simulink model "Medium_Self_Balance_Vehicle"  (R2021b)
settings: Solver=FixedStepDiscrete  StartTime=0.0  StopTime=10.0  FixedStep=0.005  RelTol=1e-3
libraries: TIMERS_Lib x9, GPIO_Lib x8, REG_Lib x4, ADC_Lib x1, STM32_Config_Lib x1, USART_Lib x1
(part 2 of 2)

== system Medium_Self_Balance_Vehicle/Function-Call Subsystem/Subsystem9/If Action Subsystem5 ==
  Action Port : ActionPort  ActionPortLabel=else { }
  Constant1 : Constant  Value=-1  OutDataTypeStr=int16
  Constant3 : Constant
  Constant4 : Constant  Value=0
  Data Store Read1 : DataStoreRead  DataStoreName=motob  IndexOptions=Index vector (dialog)  Indices=1  OutputSizes=1
  Divide : Product  Inputs=**
  GPIO_Write3 : GPIO_Lib/GPIO_Write  Port_name=GPIOB  Pin0=off  Toggle_Pin0=off  Pin1=off  Toggle_Pin1=off  Pin2=off  Toggle_Pin2=off  Pin3=off  Toggle_Pin3=off  Pin4=off  Toggle_Pin4=off  Pin5=off  Toggle_Pin5=off  Pin6=off  Toggle_Pin6=off  Pin7=off  Toggle_Pin7=off  Pin8=off  Toggle_Pin8=off  Pin9=off  Toggle_Pin9=off  Pin10=off  Toggle_Pin10=off  Pin11=off  Toggle_Pin11=off  Pin12=on  Toggle_Pin12=off  Pin13=on  Toggle_Pin13=off  Pin14=off  Toggle_Pin14=off  Pin15=off  Toggle_Pin15=off  PinList="GPIOA4  15GPIOB3   4   5   8   9  12  13  14  15"
      settings: SourceProductName=Target Support Package - STM32 Adapter
  Timers : TIMERS_Lib/Timers  currentTIM=TIM1  TIM_Name=TIM1  sysUsingTimer=off  TIM_APBClock=72000000  TIM_Set_Clk=off  TIM_Prescaler=0  TIM_Clock=72000000.00  Variable_frequency=off  TIM_Set_OutFreq=off  TIM_ARR=7199  Output_frequency=10001.39  Repetition_counter=0  TIM_Mode=Up  TIM_DMA=none  TIM_IRQ=off  TIM_IRQ_ONLY=off  TIM_UP=off  TIM_TRG=off  TIM_COM=off  TIM_BRK=off  NbTIM=4  CH1_enable=on  CH1N_enable=off  CH1_type=Output_PWM  CH1_DMA=off  CH1_int=off  CH1_edge=Rising  CH1_div=1  CH1_variable_duty=off  CH1_set_pulse=off  CH1_output_duty=0.00  CH1_pulse=0  CH2_enable=off  CH2N_enable=off  CH2_type=Unknown  CH2_DMA=off  CH2_int=off  CH2_edge=Rising  CH2_div=1  CH2_variable_duty=off  CH2_set_pulse=off  CH2_output_duty=0.00  CH2_pulse=0  CH3_enable=off  CH3N_enable=off  CH3_type=Unknown  CH3_DMA=off  CH3_int=off  CH3_edge=Rising  CH3_div=1  CH3_variable_duty=off  CH3_set_pulse=off  CH3_output_duty=0.00  CH3_pulse=0  CH4_enable=on  CH4N_enable=off  CH4_type=Output_PWM  CH4_DMA=off  CH4_int=off  CH4_edge=Rising  CH4_div=1  CH4_variable_duty=on  CH4_set_pulse=off  CH4_output_duty=0.00  CH4_pulse=0
      settings: SourceProductName=Target Support Package - STM32 Adapter
  wires:
  Constant1/1 -> Divide/2
  Data Store Read1/1 -> Divide/1
  Constant4/1 -> GPIO_Write3/1
  Divide/1 -> Timers/1
  Constant3/1 -> GPIO_Write3/2

== system Medium_Self_Balance_Vehicle/Function-Call Subsystem/Subsystem9/If Action Subsystem6 ==
  Action Port : ActionPort  ActionPortLabel=if { }
  Constant : Constant  Value=0
  Constant1 : Constant
  Data Store Read1 : DataStoreRead  DataStoreName=motob  IndexOptions=Index vector (dialog)  Indices=1  OutputSizes=1
  GPIO_Write1 : GPIO_Lib/GPIO_Write  Port_name=GPIOB  Pin0=off  Toggle_Pin0=off  Pin1=off  Toggle_Pin1=off  Pin2=off  Toggle_Pin2=off  Pin3=off  Toggle_Pin3=off  Pin4=off  Toggle_Pin4=off  Pin5=off  Toggle_Pin5=off  Pin6=off  Toggle_Pin6=off  Pin7=off  Toggle_Pin7=off  Pin8=off  Toggle_Pin8=off  Pin9=off  Toggle_Pin9=off  Pin10=off  Toggle_Pin10=off  Pin11=off  Toggle_Pin11=off  Pin12=on  Toggle_Pin12=off  Pin13=on  Toggle_Pin13=off  Pin14=off  Toggle_Pin14=off  Pin15=off  Toggle_Pin15=off  PinList="GPIOA4  15GPIOB3   4   5   8   9  12  13  14  15"
      settings: SourceProductName=Target Support Package - STM32 Adapter
  Timers : TIMERS_Lib/Timers  currentTIM=TIM1  TIM_Name=TIM1  sysUsingTimer=off  TIM_APBClock=72000000  TIM_Set_Clk=off  TIM_Prescaler=0  TIM_Clock=72000000.00  Variable_frequency=off  TIM_Set_OutFreq=off  TIM_ARR=7200  Output_frequency=10000.00  Repetition_counter=0  TIM_Mode=Up  TIM_DMA=none  TIM_IRQ=off  TIM_IRQ_ONLY=off  TIM_UP=off  TIM_TRG=off  TIM_COM=off  TIM_BRK=off  NbTIM=4  CH1_enable=on  CH1N_enable=off  CH1_type=Output_PWM  CH1_DMA=off  CH1_int=off  CH1_edge=Rising  CH1_div=1  CH1_variable_duty=off  CH1_set_pulse=off  CH1_output_duty=0.00  CH1_pulse=0  CH2_enable=off  CH2N_enable=off  CH2_type=Unknown  CH2_DMA=off  CH2_int=off  CH2_edge=Rising  CH2_div=1  CH2_variable_duty=off  CH2_set_pulse=off  CH2_output_duty=0.00  CH2_pulse=0  CH3_enable=off  CH3N_enable=off  CH3_type=Unknown  CH3_DMA=off  CH3_int=off  CH3_edge=Rising  CH3_div=1  CH3_variable_duty=off  CH3_set_pulse=off  CH3_output_duty=0.00  CH3_pulse=0  CH4_enable=on  CH4N_enable=off  CH4_type=Output_PWM  CH4_DMA=off  CH4_int=off  CH4_edge=Rising  CH4_div=1  CH4_variable_duty=on  CH4_set_pulse=off  CH4_output_duty=0.00  CH4_pulse=0
      settings: SourceProductName=Target Support Package - STM32 Adapter
  wires:
  Constant/1 -> GPIO_Write1/2
  Constant1/1 -> GPIO_Write1/1
  Data Store Read1/1 -> Timers/1

== system Medium_Self_Balance_Vehicle/Function-Call Subsystem/Subsystem5/Atomic Subsystem/If Action Subsystem ==
  Action Port : ActionPort  ActionPortLabel=if { }
  Add : Sum
  Constant : Constant  OutDataTypeStr=int16
  Data Store Read : DataStoreRead  DataStoreName=key5_flag  IndexOptions=Index vector (dialog)  Indices=1  OutputSizes=1
  Data Store Write : DataStoreWrite  DataStoreName=key5_flag  IndexOptions=Index vector (dialog)  Indices=1  OutputSizes=1
  wires:
  Data Store Read/1 -> Add/1
  Constant/1 -> Add/2
  Add/1 -> Data Store Write/1

== system Medium_Self_Balance_Vehicle/Function-Call Subsystem/Subsystem5/Atomic Subsystem/If Action Subsystem1 ==
  Action Port : ActionPort  ActionPortLabel=else { }
  Data Store Read1 : DataStoreRead  DataStoreName=key5_flag  IndexOptions=Index vector (dialog)  Indices=1  OutputSizes=1
  If : If  IfExpression=u1 >= 2
  If Action Subsystem : Subsystem  TreatAsAtomicUnit=on
  If Action Subsystem1 : Subsystem  TreatAsAtomicUnit=on
  wires:
  If/1 -> If Action Subsystem/Action
  Data Store Read1/1 -> If/1
  If/2 -> If Action Subsystem1/Action

== system Medium_Self_Balance_Vehicle/Function-Call Subsystem/Subsystem5/Atomic Subsystem/If Action Subsystem1/If Action Subsystem ==
  Action Port : ActionPort  ActionPortLabel=if { }
  Constant : Constant  OutDataTypeStr=int16
  Constant1 : Constant  Value=0  OutDataTypeStr=int16
  Data Store Write1 : DataStoreWrite  DataStoreName=key5_click  IndexOptions=Index vector (dialog)  Indices=1  OutputSizes=1
  Data Store Write2 : DataStoreWrite  DataStoreName=key5_flag  IndexOptions=Index vector (dialog)  Indices=1  OutputSizes=1
  wires:
  Constant/1 -> Data Store Write1/1
  Constant1/1 -> Data Store Write2/1

== system Medium_Self_Balance_Vehicle/Function-Call Subsystem/Subsystem5/Atomic Subsystem/If Action Subsystem1/If Action Subsystem1 ==
  Action Port : ActionPort  ActionPortLabel=else { }
  Constant : Constant  Value=0  OutDataTypeStr=int16
  Constant1 : Constant  Value=0  OutDataTypeStr=int16
  Data Store Write1 : DataStoreWrite  DataStoreName=key5_click  IndexOptions=Index vector (dialog)  Indices=1  OutputSizes=1
  Data Store Write2 : DataStoreWrite  DataStoreName=key5_flag  IndexOptions=Index vector (dialog)  Indices=1  OutputSizes=1
  wires:
  Constant/1 -> Data Store Write1/1
  Constant1/1 -> Data Store Write2/1

== stateflow chart Medium_Self_Balance_Vehicle/Function-Call Subsystem/Subsystem3/Chart ==
  (default) -> (junction 1)
  (junction 1) -> (junction 3) : {MPU6050ReadDATA(accel,Tempera,gyro);}
  data: accel output int16 size=3; Tempera output int16 size=1; gyro output int16 size=3

== matlab function Medium_Self_Balance_Vehicle/MATLAB Function ==
  data: u1 input; NbChar output; Buff output; u2 input
function [NbChar, Buff] = convert(u1,u2)
if coder.target('Sfun')
% Executing in MATLAB, Buff is null
Buff = uint32(0);
NbChar = uint16(0);
else
% Executing in the generated code. 
%buffer is an array of 15 unsigned char
buffer = zeros(1,32,'uint8');
%Generate C code using sprintf to write input value as float in buffer
coder.ceval('sprintf',coder.wref(buffer),['u1= %5d,u2= %5d',0],u1,u2);
y = [buffer(1:24),13,10,0];
%Call getBuffPtr extern C function to get pointer address of y buffer 
Buff = coder.ceval('getBuffPtr',coder.ref(y));
NbChar = uint16(size(y,2));
end
end

== stateflow chart Medium_Self_Balance_Vehicle/Chart ==
  (default) -> (junction 51) : % i
  (junction 51) -> (junction 52) [order 1] : [i<1]
  (junction 51) -> (junction 53) [order 2] : [i>=1]
  (junction 52) -> (junction 54) : {IIC_Init();MPU6050_initialize();i = i + 1;}
  (junction 54) -> (junction 53)
  (junction 53) -> (junction 55)
  data: i local double
